simulink model "state"  (R2020a)
settings: Solver=VariableStepAuto  StartTime=0.0  StopTime=100.0  RelTol=1e-3
values from neighbouring files (symbols this model uses):
  A = [((-xp0-Ks1-K0)/Cv1) , (K0/Cv1) ; ((K0+xp0)/Cv2) , ((-K0-xp0-Ks2)/Cv2)]    [Skrypt.m]    (also in proj.m)
  B = [ (xp0/Cv1) ,    (Ks1/Cv1)   ;  0,        (Ks2/Cv2)     ]    [Skrypt.m]    (also in proj.m)
  C = [1,0;0,1]    [Skrypt.m]    (also in proj.m)
  D = zeros(2)    [Skrypt.m]    (also in proj.m)
  dTkz0 = 0    [Skrypt.m]    (also in proj.m)
  dTzew0 = 0    [Skrypt.m]    (also in proj.m)
  steptime = 50    [proj.m]
  Tkz0 = TkzN    (= 30)    [Skrypt.m]    (also in proj.m)
  Tw = -(A^(-1))*B*u    [proj.m]
  Tzew0 = TzewN    (= -20)    [Skrypt.m]    (also in proj.m)
settings Model: Creator=pc  LastModifiedBy=pc

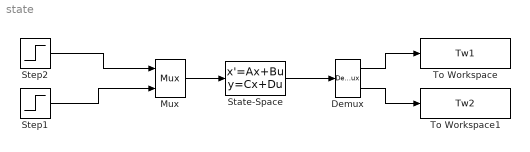
== system state ==
  Demux : Demux  Outputs=2
  Mux : Mux  Inputs=2
  State-Space : StateSpace  A=A  B=B  C=C  D=D  InitialCondition=Tw
  Step1 : Step  Time=steptime  Before=Tzew0  After=Tzew0+dTzew0  SampleTime=0
  Step2 : Step  Time=steptime  Before=Tkz0  After=Tkz0+dTkz0  SampleTime=0
  To Workspace : ToWorkspace  VariableName=Tw1  SampleTime=-1
  To Workspace1 : ToWorkspace  VariableName=Tw2  SampleTime=-1
  wires:
  Step1/1 -> Mux/2
  Demux/1 -> To Workspace/1
  State-Space/1 -> Demux/1
  Demux/2 -> To Workspace1/1
  Mux/1 -> State-Space/1
  Step2/1 -> Mux/1
